simulink model "Grid"  (R2015b)
settings: configuration reference "GridSet" (kept outside this file)
settings Model: Creator=Emilio  LastModifiedBy=Emilio
settings ConfigSetRef: SourceLocation=Base Workspace

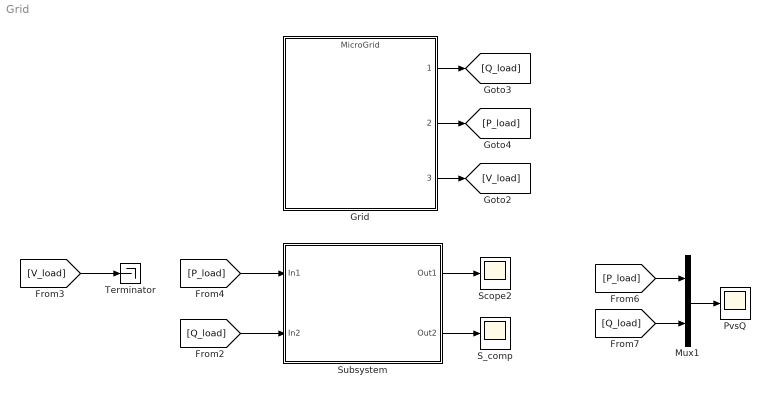
== system Grid ==
  "Grid " : ModelReference  ModelNameDialog=MicroGrid  ModelReferenceVersion=1.11  CopyOfModelName=MicroGrid
  Mux1 : Mux  Inputs=2
  PvsQ : Scope
  S_comp : Scope
  Scope2 : Scope
  Subsystem : Subsystem
  Terminator : Terminator
  wires:
  "Grid "/1 -> [Q_load]
  "Grid "/2 -> [P_load]
  "Grid "/3 -> [V_load]
  [V_load] -> Terminator/1
  Mux1/1 -> PvsQ/1
  [P_load] -> Mux1/1
  [Q_load] -> Mux1/2
  [P_load] -> Subsystem/1(In1)
  [Q_load] -> Subsystem/2(In2)
  Subsystem/1(Out1) -> Scope2/1
  Subsystem/2(Out2) -> S_comp/1

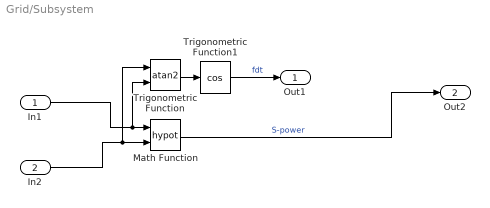
== system Grid/Subsystem ==
  In1 : Inport
  In2 : Inport  Port=2
  Math Function : Math  Operator=hypot  SaturateOnIntegerOverflow=on
  Trigonometric Function : Trigonometry  Operator=atan2
  Trigonometric Function1 : Trigonometry  Operator=cos
  Out1 : Outport
  Out2 : Outport  Port=2
  wires:
  In1/1 -> Trigonometric Function/2, Math Function/1
  Trigonometric Function1/1 -> Out1/1  "fdt"
  Trigonometric Function/1 -> Trigonometric Function1/1
  Math Function/1 -> Out2/1  "S-power"
  In2/1 -> Trigonometric Function/1, Math Function/2
